simulink model "schema_robot2015a"  (R2015a)
settings: Solver=ode45  StartTime=0.0  StopTime=10.0  RelTol=1e-3
values from neighbouring files (symbols this model uses):
  RB = struct()    [robot_numeric.m]    (also in robot_numeric_2.m)
settings Model: Creator=ygorra  LastModifiedBy=planusse
settings DataIOCC: LimitDataPoints=off  SaveFormat=Dataset
settings HardwareCC: ProdBitPerPointer=64  ProdLargestAtomicFloat=Float  ProdIntDivRoundTo=Zero  ProdEndianess=LittleEndian  ProdHWDeviceType=Specified
settings ModelReferenceCC: PropagateSignalLabelsOutOfModel=on

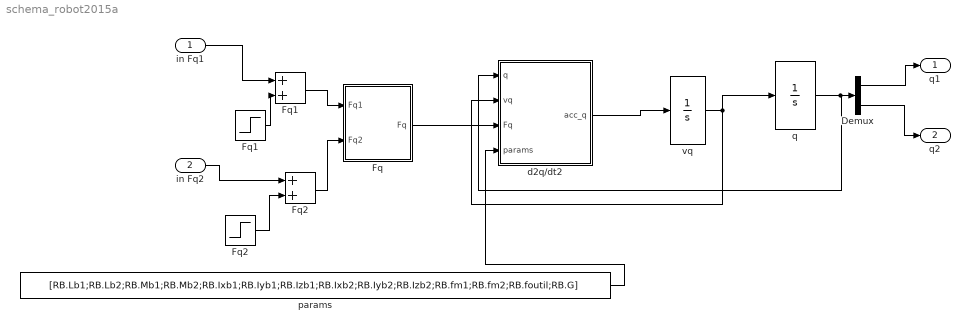
== system schema_robot2015a ==
  in Fq1 : Inport
  in Fq2 : Inport  Port=2
  Demux : Demux  Outputs=2
  Fq : MATLAB Function  TreatAsAtomicUnit=on
      settings: PermitHierarchicalResolution=ParametersOnly
  "Fq1  " : Step  Time=RB.t_Fq1  Before=RB.Fq1_0  After=RB.Fq1_1  SampleTime=0
  "Fq1   " : Sum
  "Fq2 " : Step  Time=RB.t_Fq2  Before=RB.Fq2_0  After=RB.Fq2_1  SampleTime=0
  "Fq2   " : Sum
  d2q/dt2 : MATLAB Function  TreatAsAtomicUnit=on
      settings: PermitHierarchicalResolution=ParametersOnly
  params : Constant  Value=[RB.Lb1;RB.Lb2;RB.Mb1;RB.Mb2;RB.Ixb1;RB.Iyb1;RB.Izb1;RB.Ixb2;RB.Iyb2;RB.Izb2;RB.fm1;RB.fm2;RB.foutil;RB.G]
  q : Integrator  InitialCondition=[RB.q1_init;RB.q2_init]  ContinuousStateAttributes='q'
  vq : Integrator  InitialCondition=[RB.vq1_init;RB.vq2_init]  ContinuousStateAttributes='vq'
  q1 : Outport
  q2 : Outport  Port=2
  wires:
  Demux/1 -> q1/1
  d2q/dt2/1(acc_q) -> vq/1
  vq/1 -> d2q/dt2/2(vq), q/1
  q/1 -> Demux/1, d2q/dt2/1(q)
  Fq/1(Fq) -> d2q/dt2/3(Fq)
  params/1 -> d2q/dt2/4(params)
  in Fq1/1 -> "Fq1   "/1
  "Fq1  "/1 -> "Fq1   "/2
  in Fq2/1 -> "Fq2   "/1
  "Fq2 "/1 -> "Fq2   "/2
  "Fq1   "/1 -> Fq/1(Fq1)
  "Fq2   "/1 -> Fq/2(Fq2)
  Demux/2 -> q2/1

== matlab function schema_robot2015a/Fq ==
  data: Fq1 input; Fq2 input; Fq output
function Fq=Fq_(Fq1,Fq2)
    Fq=[Fq1;Fq2];
end

== matlab function schema_robot2015a/d2q//dt2 ==
  data: q input; vq input; Fq input; acc_q output; params input
function acc_q=clc_accq(q,vq,Fq,params)
    q1=q(1);    
    q2=q(2);
    vq1=vq(1);
    vq2=vq(2);
    Lb1=params(1);
    Lb2=params(2);
    Mb1=params(3);
    Mb2=params(4);
    Ixb1=params(5);
    Iyb1=params(6);
    Izb1=params(7);
    Ixb2=params(8);
    Iyb2=params(9);
    Izb2=params(10);
    fm1=params(11);
    fm2=params(12);
    foutil=params(13);
    G=params(14);
    A= clc_A(q1,q2,Lb1,Lb2,Mb1,Mb2,Ixb1,Iyb1,Izb1,Ixb2,Iyb2,Izb2,fm1,fm2,foutil,G);
    H= clc_H(q1,q2,vq1,vq2,Lb1,Lb2,Mb1,Mb2,Ixb1,Iyb1,Izb1,Ixb2,Iyb2,Izb2,fm1,fm2,foutil,G);
    acc_q=pinv(A)*(Fq-H);
end
